simulink subsystem "NoFuelCell"  (R2023b)
settings: Solver=VariableStepAuto  StartTime=0.0  StopTime=10.0  RelTol=1e-3
settings Model: Creator=The MathWorks, Inc.  LastModifiedBy=The MathWorks, Inc.

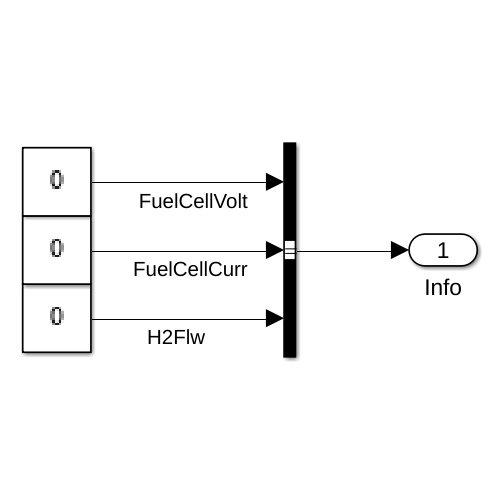
[thumbnail: Simulink's stored preview of the top-level diagram]
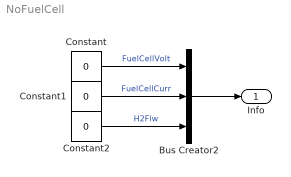
== system NoFuelCell ==
  Bus Creator2 : BusCreator  Inputs=3
  Constant : Constant  Value=0  SampleTime=-1
  Constant1 : Constant  Value=0  SampleTime=-1
  Constant2 : Constant  Value=0  SampleTime=-1
  Info : Outport
  wires:
  Bus Creator2/1 -> Info/1
  Constant1/1 -> Bus Creator2/2  "FuelCellCurr"
  Constant/1 -> Bus Creator2/1  "FuelCellVolt"
  Constant2/1 -> Bus Creator2/3  "H2Flw"
